simulink model "npc_controller"  (R2022a)
settings: Solver=FixedStepDiscrete  StartTime=0.0  StopTime=20  RelTol=1e-3  EnableMultiTasking=on
undefined symbols (not defined in the file): CAN_O_INT, CANA_BASE, Down, GPTRIP1SEL, GPTRIP2SEL, GPTRIP3SEL, Tsw, TZ1, TZ2, TZ3, Up, V2G_en
libraries: simulink x171, hdlsllib x90, c2802xlib x46, c2837xDlib x19, c280xlib x12, canmsglib x9, c2838xlib x8, idelinklib_common x5, c2806xlib x2, slpidlib x2, c28004xlib x2, c281xlib x2
(part 38 of 55)

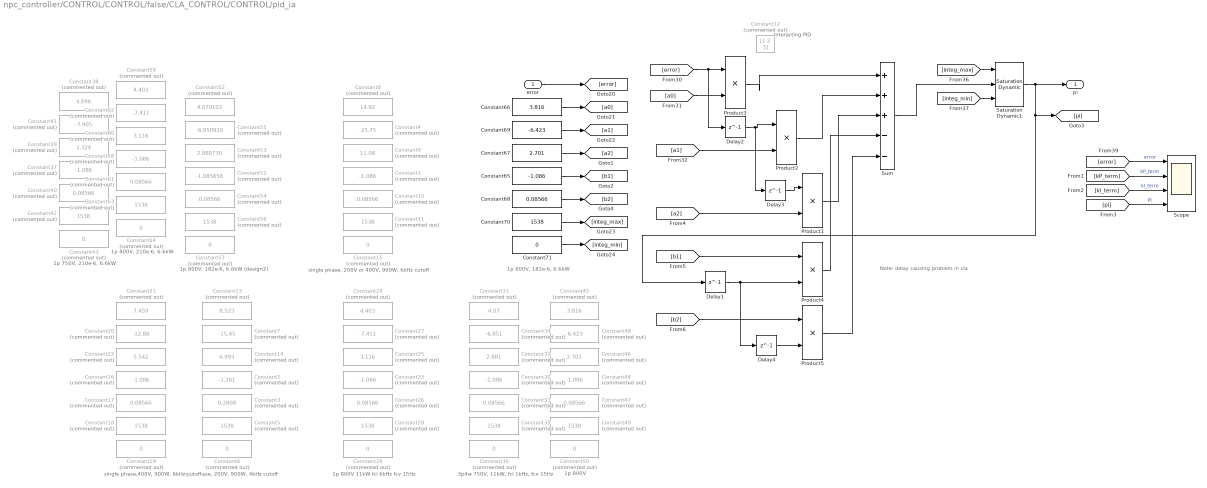
== system npc_controller/CONTROL/CONTROL/false/CLA_CONTROL/CONTROL/pid_ia ==
  note: single phase, 200V or 400V, 900W, 6kHz cutoff
  note: interacting PID
  note: Note: delay causing problem in cla
  note: single phase, 200V, 900W, 4kHz cutoff
  note: single phase,400V, 900W, 6kHz cutoff
  note: 1p 800V 11kW fci 6kHz fcv 15Hz
  note: 3p4w 750V, 11kW, fci 1kHz, fcv 15Hz
  note: 1p 750V, 210e-6, 6.6kW
  note: 1p 800V
  note: 1p 800V, 182e-6, 6.6kW (design2)
  note: 1p 800V, 210e-6, 6.6kW
  note: 1p 800V, 182e-6, 6.6kW
  error : Inport  OutDataTypeStr=single
  Constant{1,16,23,30,37,44,58} (7 alike) : Constant  Commented=on  Value=-1.086  OutDataTypeStr=single
  Constant{10,17,26,33,40,47,54,61} (8 alike) : Constant  Commented=on  Value=0.08566  OutDataTypeStr=single
  Constant{5,11,18,28,35,42,49,56,63} (9 alike) : Constant  Commented=on  Value=1538  OutDataTypeStr=single
  Constant12 : Constant  Commented=on  Value=[1 2 3]  OutDataTypeStr=single
  Constant13 : Constant  Commented=on  Value=8.523  VectorParams1D=off  OutDataTypeStr=single
  Constant14 : Constant  Commented=on  Value=6.993  OutDataTypeStr=single
  Constant{6,15,19,29,36,43,50,57,64} (9 alike) : Constant  Commented=on  Value=0  OutDataTypeStr=single
  Constant2 : Constant  Commented=on  Value=-1.281  OutDataTypeStr=single
  Constant20 : Constant  Commented=on  Value=-12.88  OutDataTypeStr=single
  Constant21 : Constant  Commented=on  Value=7.459  VectorParams1D=off  OutDataTypeStr=single
  Constant22 : Constant  Commented=on  Value=5.542  OutDataTypeStr=single
  Constant24 : Constant  Commented=on  Value=4.403  VectorParams1D=off  OutDataTypeStr=single
  Constant25 : Constant  Commented=on  Value=3.116  OutDataTypeStr=single
  Constant27 : Constant  Commented=on  Value=-7.411  OutDataTypeStr=single
  Constant3 : Constant  Commented=on  Value=0.2808  OutDataTypeStr=single
  Constant31 : Constant  Commented=on  Value=4.07  VectorParams1D=off  OutDataTypeStr=single
  Constant32 : Constant  Commented=on  Value=2.881  OutDataTypeStr=single
  Constant34 : Constant  Commented=on  Value=-6.851  OutDataTypeStr=single
  Constant38 : Constant  Commented=on  Value=4.696  VectorParams1D=off  OutDataTypeStr=single
  Constant39 : Constant  Commented=on  Value=3.324  OutDataTypeStr=single
  Constant4 : Constant  Commented=on  Value=-25.75  OutDataTypeStr=single
  Constant41 : Constant  Commented=on  Value=-7.905  OutDataTypeStr=single
  Constant45 : Constant  Commented=on  Value=3.816  VectorParams1D=off  OutDataTypeStr=single
  Constant46 : Constant  Commented=on  Value=2.701  OutDataTypeStr=single
  Constant48 : Constant  Commented=on  Value=-6.423  OutDataTypeStr=single
  Constant51 : Constant  Commented=on  Value=-1.085658  OutDataTypeStr=single
  Constant52 : Constant  Commented=on  Value=4.070103  VectorParams1D=off  OutDataTypeStr=single
  Constant53 : Constant  Commented=on  Value=2.880730  OutDataTypeStr=single
  Constant55 : Constant  Commented=on  Value=-6.850920  OutDataTypeStr=single
  Constant59 : Constant  Commented=on  Value=4.403  VectorParams1D=off  OutDataTypeStr=single
  Constant60 : Constant  Commented=on  Value=3.116  OutDataTypeStr=single
  Constant62 : Constant  Commented=on  Value=-7.411  OutDataTypeStr=single
  Constant65 : Constant  Value=-1.086  OutDataTypeStr=single
  Constant66 : Constant  Value=3.816  VectorParams1D=off  OutDataTypeStr=single
  Constant67 : Constant  Value=2.701  OutDataTypeStr=single
  Constant68 : Constant  Value=0.08566  OutDataTypeStr=single
  Constant69 : Constant  Value=-6.423  OutDataTypeStr=single
  Constant7 : Constant  Commented=on  Value=-15.45  OutDataTypeStr=single
  Constant70 : Constant  Value=1538  OutDataTypeStr=single
  Constant71 : Constant  Value=0  OutDataTypeStr=single
  Constant8 : Constant  Commented=on  Value=14.92  VectorParams1D=off  OutDataTypeStr=single
  Constant9 : Constant  Commented=on  Value=11.08  OutDataTypeStr=single
  Delay1 : Delay  DelayLength=1  InitialCondition=0  StateName=ia_pid3  StateMustResolveToSignalObject=on
  Delay2 : Delay  DelayLength=1  InitialCondition=0  StateName=ia_pid1  StateMustResolveToSignalObject=on
  Delay3 : Delay  DelayLength=1  InitialCondition=0  StateName=ia_pid2  StateMustResolveToSignalObject=on
  Delay4 : Delay  DelayLength=1  InitialCondition=0  StateName=ia_pid4  StateMustResolveToSignalObject=on
  Product{1..5} (5 alike) : Product  OutDataTypeStr=single
  Saturation Dynamic1 : simulink/Discontinuities/Saturation Dynamic  OutMin=[]  OutMax=[]  OutDataTypeStr=single  OutputDataTypeScalingMode=single  OutDataType=fixdt(1, 16)  OutScaling=2^-10  DoSatur=off
  Scope : Scope  NumInputPorts=4
  Sum : Sum  Inputs=|+++--  AccumDataTypeStr=single  OutDataTypeStr=single
  pi : Outport
  wires:
  Constant68/1 -> [b2]
  Constant67/1 -> [a2]
  Constant65/1 -> [b1]
  [b2] -> Product5/1
  Product4/1 -> Sum/4
  Product5/1 -> Sum/5
  Delay4/1 -> Product5/2
  [b1] -> Product4/1
  Delay1/1 -> Delay4/1, Product4/2
  Product1/1 -> Sum/3
  Product2/1 -> Sum/2
  Product3/1 -> Sum/1
  [a2] -> Product1/2
  Delay3/1 -> Product1/1
  Saturation Dynamic1/1 -> [pi], Delay1/1, pi/1
  Delay2/1 -> Delay3/1, Product2/1
  [error] -> Product3/1, Delay2/1
  Constant66/1 -> [a0]
  [a1] -> Product2/2
  error/1 -> [error]
  Constant69/1 -> [a1]
  Constant71/1 -> [integ_min]
  Constant70/1 -> [integ_max]
  [integ_max] -> Saturation Dynamic1/1
  [integ_min] -> Saturation Dynamic1/3
  Sum/1 -> Saturation Dynamic1/2
  [a0] -> Product3/2
  [pi] -> Scope/4  "PI"
  [kI_term] -> Scope/3  "kI_term"
  [kP_term] -> Scope/2  "kP_term"
  [error] -> Scope/1  "error"

== system npc_controller/CONTROL/CONTROL/false/CLA_CONTROL/CONTROL/pid_ib ==
  note: Note: delay causing problem in cla
  note: interacting PID
  note: 1p 800V, 182e-6, 6.6kW
  note: single phase, 200V or 400V, 900W, 6kHz cutoff
  note: 1p 800V, 182e-6, 6.6kW (design2)
  error : Inport  OutDataTypeStr=single
  Constant1 : Constant  Commented=on  Value=-1.086  OutDataTypeStr=single
  Constant10 : Constant  Commented=on  Value=0.08566  OutDataTypeStr=single
  Constant11 : Constant  Commented=on  Value=1538  OutDataTypeStr=single
  Constant12 : Constant  Commented=on  Value=[1 2 3]  OutDataTypeStr=single
  Constant13 : Constant  Commented=on  Value=1538  OutDataTypeStr=single
  Constant14 : Constant  Commented=on  Value=0  OutDataTypeStr=single
  Constant15 : Constant  Commented=on  Value=0  OutDataTypeStr=single
  Constant2 : Constant  Commented=on  Value=-1.085658  OutDataTypeStr=single
  Constant3 : Constant  Commented=on  Value=4.070103  VectorParams1D=off  OutDataTypeStr=single
  Constant4 : Constant  Commented=on  Value=-25.75  OutDataTypeStr=single
  Constant5 : Constant  Commented=on  Value=2.880730  OutDataTypeStr=single
  Constant51 : Constant  Value=-1.086  OutDataTypeStr=single
  Constant52 : Constant  Value=3.816  VectorParams1D=off  OutDataTypeStr=single
  Constant53 : Constant  Value=2.701  OutDataTypeStr=single
  Constant54 : Constant  Value=0.08566  OutDataTypeStr=single
  Constant55 : Constant  Value=-6.423  OutDataTypeStr=single
  Constant56 : Constant  Value=1538  OutDataTypeStr=single
  Constant57 : Constant  Value=0  OutDataTypeStr=single
  Constant6 : Constant  Commented=on  Value=0.08566  OutDataTypeStr=single
  Constant7 : Constant  Commented=on  Value=-6.850920  OutDataTypeStr=single
  Constant8 : Constant  Commented=on  Value=14.92  VectorParams1D=off  OutDataTypeStr=single
  Constant9 : Constant  Commented=on  Value=11.08  OutDataTypeStr=single
  Delay1 : Delay  DelayLength=1  InitialCondition=0  StateName=ib_pid3  StateMustResolveToSignalObject=on
  Delay2 : Delay  DelayLength=1  InitialCondition=0  StateName=ib_pid1  StateMustResolveToSignalObject=on
  Delay3 : Delay  DelayLength=1  InitialCondition=0  StateName=ib_pid2  StateMustResolveToSignalObject=on
  Delay4 : Delay  DelayLength=1  InitialCondition=0  StateName=ib_pid4  StateMustResolveToSignalObject=on
  Product{1..5} (5 alike) : Product  OutDataTypeStr=single
  Saturation Dynamic1 : simulink/Discontinuities/Saturation Dynamic  OutMin=[]  OutMax=[]  OutDataTypeStr=single  OutputDataTypeScalingMode=single  OutDataType=fixdt(1, 16)  OutScaling=2^-10  DoSatur=off
  Scope : Scope  NumInputPorts=4
  Sum : Sum  Inputs=|+++--  AccumDataTypeStr=single  OutDataTypeStr=single
  pi : Outport
  wires:
  [error] -> Scope/1  "error"
  [kP_term] -> Scope/2  "kP_term"
  [kI_term] -> Scope/3  "kI_term"
  [pi] -> Scope/4  "PI"
  [a0] -> Product3/2
  Sum/1 -> Saturation Dynamic1/2
  [integ_min] -> Saturation Dynamic1/3
  [integ_max] -> Saturation Dynamic1/1
  error/1 -> [error]
  [a1] -> Product2/2
  [error] -> Delay2/1, Product3/1
  Delay2/1 -> Product2/1, Delay3/1
  Saturation Dynamic1/1 -> pi/1, Delay1/1, [pi]
  Delay3/1 -> Product1/1
  [a2] -> Product1/2
  Product3/1 -> Sum/1
  Product2/1 -> Sum/2
  Product1/1 -> Sum/3
  Delay1/1 -> Product4/2, Delay4/1
  [b1] -> Product4/1
  Delay4/1 -> Product5/2
  Product5/1 -> Sum/5
  Product4/1 -> Sum/4
  [b2] -> Product5/1
  Constant52/1 -> [a0]
  Constant55/1 -> [a1]
  Constant53/1 -> [a2]
  Constant51/1 -> [b1]
  Constant54/1 -> [b2]
  Constant56/1 -> [integ_max]
  Constant57/1 -> [integ_min]

== system npc_controller/CONTROL/CONTROL/false/CLA_CONTROL/CONTROL/pid_ic ==
  note: interacting PID
  note: Note: delay causing problem in cla
  note: 1p 800V, 182e-6, 6.6kW
  note: single phase, 200V or 400V, 900W, 6kHz cutoff
  note: 1p 800V, 182e-6, 6.6kW (design2)
  error : Inport  OutDataTypeStr=single
  Constant1 : Constant  Commented=on  Value=-1.086  OutDataTypeStr=single
  Constant10 : Constant  Commented=on  Value=0.08566  OutDataTypeStr=single
  Constant11 : Constant  Commented=on  Value=1538  OutDataTypeStr=single
  Constant12 : Constant  Commented=on  Value=[1 2 3]  OutDataTypeStr=single
  Constant13 : Constant  Commented=on  Value=1538  OutDataTypeStr=single
  Constant14 : Constant  Commented=on  Value=0  OutDataTypeStr=single
  Constant15 : Constant  Commented=on  Value=0  OutDataTypeStr=single
  Constant2 : Constant  Commented=on  Value=-1.085658  OutDataTypeStr=single
  Constant3 : Constant  Commented=on  Value=4.070103  VectorParams1D=off  OutDataTypeStr=single
  Constant4 : Constant  Commented=on  Value=-25.75  OutDataTypeStr=single
  Constant5 : Constant  Commented=on  Value=2.880730  OutDataTypeStr=single
  Constant51 : Constant  Value=-1.086  OutDataTypeStr=single
  Constant52 : Constant  Value=3.816  VectorParams1D=off  OutDataTypeStr=single
  Constant53 : Constant  Value=2.701  OutDataTypeStr=single
  Constant54 : Constant  Value=0.08566  OutDataTypeStr=single
  Constant55 : Constant  Value=-6.423  OutDataTypeStr=single
  Constant56 : Constant  Value=1538  OutDataTypeStr=single
  Constant57 : Constant  Value=0  OutDataTypeStr=single
  Constant6 : Constant  Commented=on  Value=0.08566  OutDataTypeStr=single
  Constant7 : Constant  Commented=on  Value=-6.850920  OutDataTypeStr=single
  Constant8 : Constant  Commented=on  Value=14.92  VectorParams1D=off  OutDataTypeStr=single
  Constant9 : Constant  Commented=on  Value=11.08  OutDataTypeStr=single
  Delay1 : Delay  DelayLength=1  InitialCondition=0  StateName=ic_pid3  StateMustResolveToSignalObject=on
  Delay2 : Delay  DelayLength=1  InitialCondition=0  StateName=ic_pid1  StateMustResolveToSignalObject=on
  Delay3 : Delay  DelayLength=1  InitialCondition=0  StateName=ic_pid2  StateMustResolveToSignalObject=on
  Delay4 : Delay  DelayLength=1  InitialCondition=0  StateName=ic_pid4  StateMustResolveToSignalObject=on
  Product{1..5} (5 alike) : Product  OutDataTypeStr=single
  Saturation Dynamic1 : simulink/Discontinuities/Saturation Dynamic  OutMin=[]  OutMax=[]  OutDataTypeStr=single  OutputDataTypeScalingMode=single  OutDataType=fixdt(1, 16)  OutScaling=2^-10  DoSatur=off
  Scope : Scope  NumInputPorts=4
  Sum : Sum  Inputs=|+++--  AccumDataTypeStr=single  OutDataTypeStr=single
  pi : Outport
  wires:
  Constant54/1 -> [b2]
  Constant53/1 -> [a2]
  Constant51/1 -> [b1]
  [b2] -> Product5/1
  Product4/1 -> Sum/4
  Product5/1 -> Sum/5
  Delay4/1 -> Product5/2
  [b1] -> Product4/1
  Delay1/1 -> Delay4/1, Product4/2
  Product1/1 -> Sum/3
  Product2/1 -> Sum/2
  Product3/1 -> Sum/1
  [a2] -> Product1/2
  Delay3/1 -> Product1/1
  Saturation Dynamic1/1 -> [pi], Delay1/1, pi/1
  Delay2/1 -> Delay3/1, Product2/1
  [error] -> Product3/1, Delay2/1
  Constant52/1 -> [a0]
  [a1] -> Product2/2
  error/1 -> [error]
  Constant55/1 -> [a1]
  Constant57/1 -> [integ_min]
  Constant56/1 -> [integ_max]
  [integ_max] -> Saturation Dynamic1/1
  [integ_min] -> Saturation Dynamic1/3
  Sum/1 -> Saturation Dynamic1/2
  [a0] -> Product3/2
  [pi] -> Scope/4  "PI"
  [kI_term] -> Scope/3  "kI_term"
  [kP_term] -> Scope/2  "kP_term"
  [error] -> Scope/1  "error"
